simulink model "TRDP_head_pack"  (R2021a)
settings: configuration reference "ART_1G_IDS_Speedgoat" (kept outside this file)
libraries: commutil2 x22, etargetslib x2, simulink x2
settings Model: DataDictionary=Model_Config.sldd  Creator=xinrui  LastModifiedBy=xinrui
settings ConfigSetRef: SourceName=ART_1G_IDS_Speedgoat

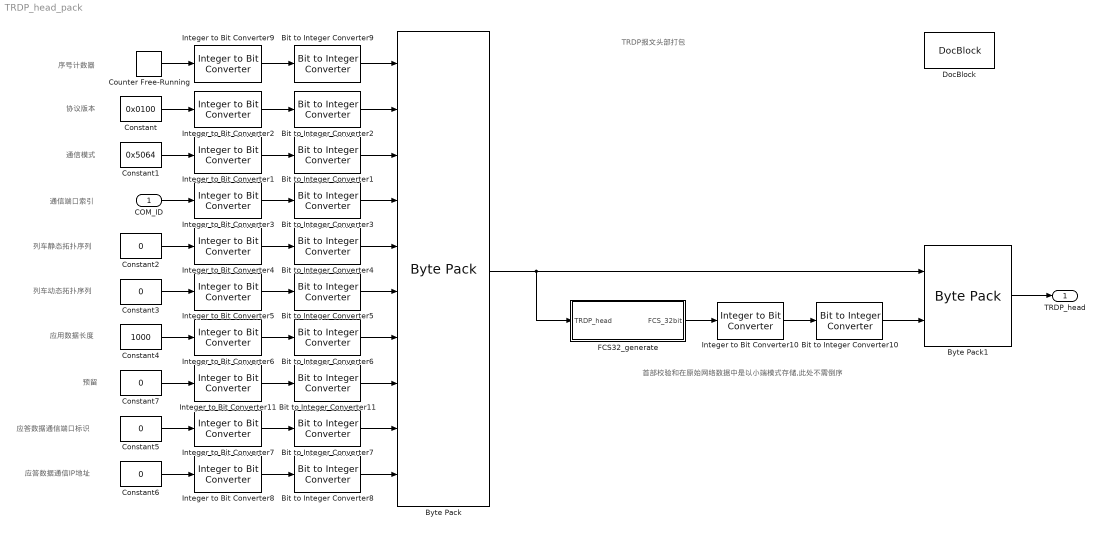
== system TRDP_head_pack ==
  note: 协议版本
  note: 通信模式
  note: 通信端口索引
  note: 列车静态拓扑序列
  note: 列车动态拓扑序列
  note: 应用数据长度
  note: 应答数据通信端口标识
  note: 应答数据通信IP地址
  note: 序号计数器
  note: 首部校验和在原始网络数据中是以小端模式存储,此处不需倒序
  note: 预留
  note: TRDP报文头部打包
  COM_ID : Inport  OutDataTypeStr=uint32  PortDimensions=1
  Bit to Integer Converter{1..9,11} (10 alike) : commutil2/Bit to Integer Converter  nbits=8  bitOrder=MSB first  signedOutputValues=Unsigned  outDtype=uint8  outDtypeSigned=Inherit via internal rule
  Bit to Integer Converter10 : commutil2/Bit to Integer Converter  nbits=8  bitOrder=LSB first  signedOutputValues=Unsigned  outDtype=uint8  outDtypeSigned=Inherit via internal rule
  Byte Pack : etargetslib/Byte Pack  datatypes={'uint8','uint8','uint8','uint8','uint8','uint8','uint8','uint8','uint8','uint8'}  byteAlign=1
  Byte Pack1 : etargetslib/Byte Pack  datatypes={'uint8','uint8'}  byteAlign=1
  Constant : Constant  Value=0x0100  OutDataTypeStr=uint16  SampleTime=-1
  Constant1 : Constant  Value=0x5064  OutDataTypeStr=uint16  SampleTime=-1
  Constant{2..3,5..7} (5 alike) : Constant  Value=0  OutDataTypeStr=uint32  SampleTime=-1
  Constant4 : Constant  Value=1000  OutDataTypeStr=uint32  SampleTime=-1
  Counter Free-Running : simulink/Sources/Counter Free-Running  NumBits=32  tsamp=-1
  DocBlock : simulink/Model-Wide Utilities/DocBlock  DocumentType=HTML  mask(DocBlock){}
      mask Display:
      | plot([.8 0 0 1 1 .8 .8 1],[1 1 0 0 .8 1 .8 .8]);
      | text(.5,.6,'CHANGELOG','horizontalalignment','center');
      | text(.95,.05,get_param(gcb,'DocumentType'),'verticalalignment','bottom','horizontalalignment','right');
  FCS32_generate : MATLAB Function  TreatAsAtomicUnit=on
  Integer to Bit Converter1 : commutil2/Integer to Bit Converter  nbits=16  signedInputValues=Unsigned  bitOrder=MSB first  outDtype=Inherit via internal rule
  Integer to Bit Converter10 : commutil2/Integer to Bit Converter  nbits=32  signedInputValues=Unsigned  bitOrder=LSB first  outDtype=Inherit via internal rule
  Integer to Bit Converter{3..9,11} (8 alike) : commutil2/Integer to Bit Converter  nbits=32  signedInputValues=Unsigned  bitOrder=MSB first  outDtype=Inherit via internal rule
  Integer to Bit Converter2 : commutil2/Integer to Bit Converter  nbits=16  signedInputValues=Unsigned  bitOrder=MSB first  outDtype=Inherit via internal rule
  TRDP_head : Outport  OutDataTypeStr=uint8  PortDimensions=40
  wires:
  Integer to Bit Converter2/1 -> Bit to Integer Converter2/1
  Constant/1 -> Integer to Bit Converter2/1
  Constant1/1 -> Integer to Bit Converter1/1
  Integer to Bit Converter1/1 -> Bit to Integer Converter1/1
  Integer to Bit Converter3/1 -> Bit to Integer Converter3/1
  COM_ID/1 -> Integer to Bit Converter3/1
  Integer to Bit Converter4/1 -> Bit to Integer Converter4/1
  Constant2/1 -> Integer to Bit Converter4/1
  Constant3/1 -> Integer to Bit Converter5/1
  Integer to Bit Converter5/1 -> Bit to Integer Converter5/1
  Integer to Bit Converter6/1 -> Bit to Integer Converter6/1
  Constant4/1 -> Integer to Bit Converter6/1
  Integer to Bit Converter8/1 -> Bit to Integer Converter8/1
  Constant6/1 -> Integer to Bit Converter8/1
  Constant5/1 -> Integer to Bit Converter7/1
  Integer to Bit Converter7/1 -> Bit to Integer Converter7/1
  Counter Free-Running/1 -> Integer to Bit Converter9/1
  Integer to Bit Converter9/1 -> Bit to Integer Converter9/1
  Bit to Integer Converter11/1 -> Byte Pack/8
  Bit to Integer Converter9/1 -> Byte Pack/1
  Bit to Integer Converter2/1 -> Byte Pack/2
  Bit to Integer Converter1/1 -> Byte Pack/3
  Bit to Integer Converter3/1 -> Byte Pack/4
  Bit to Integer Converter4/1 -> Byte Pack/5
  Bit to Integer Converter5/1 -> Byte Pack/6
  Bit to Integer Converter6/1 -> Byte Pack/7
  Bit to Integer Converter7/1 -> Byte Pack/9
  Bit to Integer Converter8/1 -> Byte Pack/10
  Integer to Bit Converter10/1 -> Bit to Integer Converter10/1
  FCS32_generate/1(FCS_32bit) -> Integer to Bit Converter10/1
  Byte Pack1/1 -> TRDP_head/1
  Byte Pack/1 -> Byte Pack1/1, FCS32_generate/1(TRDP_head)
  Bit to Integer Converter10/1 -> Byte Pack1/2
  Integer to Bit Converter11/1 -> Bit to Integer Converter11/1
  Constant7/1 -> Integer to Bit Converter11/1

== matlab function TRDP_head_pack/FCS32_generate ==
  data: TRDP_head input uint8 size=36; FCS_32bit output uint32 size=1
% 首部校验和生成
function FCS_32bit = FCS32_generate(TRDP_head)
%   1.输入参数：
%       (1)TRDP_head    TRDP头部数据
%   2.输出参数：
%       (1)FCS_32bit    计算生成的首部校验和

% 调用计算公式求解首部校验和，参与计算的原始数据为TRDP头部数据前36个字节
FCS_32bit = FCS32_calculate(TRDP_head, 36);

end
